simulink model "IEEE_1547_Testing"  (Simulink 9.2)
settings: Solver=ode4  StartTime=0.0  StopTime=inf  FixedStep=Ts  RelTol=1e-3  EnableMultiTasking=on
PreLoadFcn:
  | init_sandia
PostLoadFcn:
  | init_sandia
InitFcn:
  | init_sandia
values from neighbouring files (symbols this model uses):
  CURRENT_INPUT_OFFSET_PHA = 0    [init.m]    (also in init_sandia.m = 0.010681; init_sandia_hv.m = 0.010681)
  CURRENT_INPUT_OFFSET_PHB = 0    [init.m]    (also in init_sandia.m = 0.002978; init_sandia_hv.m = 0.002978)
  CURRENT_INPUT_OFFSET_PHC = 0    [init.m]    (also in init_sandia.m = 0.016506; init_sandia_hv.m = 0.016506)
  CURRENT_INPUT_SCALE_PHA = (1/0.03)*1.0002    (= 33.34)    [init.m]    (also in init_sandia.m = 93.940301; init_sandia_hv.m = 93.940301)
  CURRENT_INPUT_SCALE_PHB = (1/0.03)*0.9994    (= 33.3133333333)    [init.m]    (also in init_sandia.m = 94.382594; init_sandia_hv.m = 94.382594)
  CURRENT_INPUT_SCALE_PHC = (1/0.03)*0.9977    (= 33.2566666667)    [init.m]    (also in init_sandia.m = 93.670072; init_sandia_hv.m = 93.670072)
  ENABLE_PHA = 1    [init.m]    (also in init_sandia.m; init_sandia_hv.m)
  ENABLE_PHB = 1    [init.m]    (also in init_sandia.m; init_sandia_hv.m)
  ENABLE_PHC = 1    [init.m]    (also in init_sandia.m; init_sandia_hv.m)
  FNOM = 60.0    (= 60)    [init.m]    (also in init_sandia.m; init_sandia_hv.m)
  FREQUENCY = 60.0    (= 60)    [init.m]    (also in init_sandia.m; init_sandia_hv.m)
  FREQUENCY_MAX_LIMIT = 66.0    (= 66)    [init.m]    (also in init_sandia.m; init_sandia_hv.m)
  FREQUENCY_MIN_LIMIT = 56.0    (= 56)    [init.m]    (also in init_sandia.m; init_sandia_hv.m)
  FRT_CONDITION = [1 1 1 0 ]    [init.m]    (also in init_sandia.m; init_sandia_hv.m)
  FRT_END_TIMING = [0.2 0.3 0.4 0.5]    [init.m]    (also in init_sandia.m; init_sandia_hv.m)
  FRT_START_TIMING = [0.1 0.2 0.3 0.4]    [init.m]    (also in init_sandia.m; init_sandia_hv.m)
  FRT_VALUES = [59.0 56.0 55.0 33.0]    [init.m]    (also in init_sandia.m; init_sandia_hv.m)
  MODE = 1    [init.m]    (also in init_sandia.m = 3; init_sandia_hv.m = 3)
  PHASE_PHA = 0    [init_sandia.m]    (also in init_sandia_hv.m)
  PHASE_PHB = -120    [init_sandia.m]    (also in init_sandia_hv.m)
  PHASE_PHC = 120    [init_sandia.m]    (also in init_sandia_hv.m)
  RMS_ENABLE = 0    [init.m]    (also in init_sandia.m; init_sandia_hv.m)
  ROCOF_ENABLE = 0    [init.m]    (also in init_sandia.m; init_sandia_hv.m)
  ROCOF_INIT = 60    [init.m]    (also in init_sandia.m; init_sandia_hv.m)
  ROCOF_VALUE = 3    [init.m]    (also in init_sandia.m; init_sandia_hv.m)
  ROCOM_ENABLE = 1    [init.m]    (also in init_sandia.m; init_sandia_hv.m)
  ROCOM_END_TIME = 100    [init.m]    (also in init_sandia.m; init_sandia_hv.m)
  ROCOM_INIT = 1    [init.m]    (also in init_sandia.m; init_sandia_hv.m)
  ROCOM_START_TIME = 0    [init.m]    (also in init_sandia.m; init_sandia_hv.m)
  ROCOM_VALUE = 13.8    [init.m]    (also in init_sandia.m; init_sandia_hv.m)
  Ts = 40e-6    (= 4e-05)    [init.m]    (also in init_sandia.m; init_sandia_hv.m)
  VNOM = 1.0    (= 1)    [init.m]    (also in init_sandia.m = 277.2; init_sandia_hv.m = 277.2)
  VOLT_INPUT_OFFSET_PHA = 0    [init.m]    (also in init_sandia.m = 0.034058; init_sandia_hv.m = 0.034058)
  VOLT_INPUT_OFFSET_PHB = 0    [init.m]    (also in init_sandia.m = 0.06754; init_sandia_hv.m = 0.06754)
  VOLT_INPUT_OFFSET_PHC = 0    [init.m]    (also in init_sandia.m = 0.037741; init_sandia_hv.m = 0.037741)
  VOLT_INPUT_SCALE_PHA = 20    [init.m]    (also in init_sandia.m = 509.604013; init_sandia_hv.m = 509.604013)
  VOLT_INPUT_SCALE_PHB = 20    [init.m]    (also in init_sandia.m = 499.19708; init_sandia_hv.m = 499.19708)
  VOLT_INPUT_SCALE_PHC = 20    [init.m]    (also in init_sandia.m = 498.302881; init_sandia_hv.m = 498.302881)
  VOLT_OUTPUT_SCALE_PHA = 120.0*sqrt(2)    [init.m]    (also in init_sandia.m = 0.0235682300259; init_sandia_hv.m = 0.011784115013)
  VOLT_OUTPUT_SCALE_PHB = 120.0*sqrt(2)    [init.m]    (also in init_sandia.m = 0.0235682300259; init_sandia_hv.m = 0.011784115013)
  VOLT_OUTPUT_SCALE_PHC = 120.0*sqrt(2)    [init.m]    (also in init_sandia.m = 0.0235682300259; init_sandia_hv.m = 0.011784115013)
  VOLT_PHA = 1    [init_sandia.m]    (also in init_sandia_hv.m)
  VOLT_PHB = 1    [init_sandia.m]    (also in init_sandia_hv.m)
  VOLT_PHC = 1    [init_sandia.m]    (also in init_sandia_hv.m)
  VOLTAGE_MAX_LIMIT = 1.1    [init.m]    (also in init_sandia.m; init_sandia_hv.m = 1.2)
  VOLTAGE_MIN_LIMIT = 0.0    (= 0)    [init.m]    (also in init_sandia.m; init_sandia_hv.m)
  VRT_CONDITION = [0 1 0 1 0 1 0 1 -1 -1 -1 -1 -1 -1 -1 -1 -1 -1 -1 -1]+1    [init.m]    (also in init_sandia.m; init_sandia_hv.m)
  VRT_END_TIMING = [0.2 0.3 0.4 0.5 0.6 0.7 0.8 0.9 1 1.1 1.2 1.3 1.4 1.5 1.6 1.7 1.8 1.9 2 2.1]    [init.m]    (also in init_sandia.m; init_sandia_hv.m)
  VRT_PHA_ENABLE = 0    [init.m]    (also in init_sandia.m; init_sandia_hv.m)
  VRT_PHB_ENABLE = 0    [init.m]    (also in init_sandia.m; init_sandia_hv.m)
  VRT_PHC_ENABLE = 0    [init.m]    (also in init_sandia.m; init_sandia_hv.m)
  VRT_START_TIMING = [0.1 0.2 0.3 0.4 0.5 0.6 0.7 0.8 0.9 1 0.1 0.2 0.3 0.4 0.5 0.6 0.7 0.8 0.9 1]    [init.m]    (also in init_sandia.m; init_sandia_hv.m)
  VRT_VALUES = [1.2 0.94 0 0.5 0.7 0.88 0.94 0.88 0.94 1.1 1.2 0.94 0 0.5 0.7 0.88 0.94 0.88 0.94 1.1]    [init.m]    (also in init_sandia.m = [1.0 0.94 0 0.5 0.7 0.88 0.94 0.88 0.94 1.1 1.2 0.94 0 0.5 0; init_sandia_hv.m = [1.0 0.94 0 0.5 0.7 0.88 0.94 0.88 0.94 1.1 1.2 0.94 0 0.5 0)
  WAV_ENABLE = 1    [init.m]    (also in init_sandia.m; init_sandia_hv.m)
undefined symbols (not defined in the file or in its folder): DiscIntNeverNeededParam, magnitude
libraries: simulink x17, powerlib_meascontrol x13, rtlab x5, pePowerMeasurement x3, rtio_opalrt_common x3, powerlib x1
(part 1 of 2)
settings Model: ARTEMISmethode_block_infos=$$__separator__$$  Creator=DETLDAQ  LastModifiedBy=DETLDAQ  NumberOfSteps=10
settings DataIOCC: SignalLoggingSaveFormat=Dataset
settings OptimizationCC: BlockReduction=off  BooleanDataType=off  OptimizeBlockIOStorage=off  BufferReuse=off  GlobalBufferReuse=off  ExpressionFolding=off  LocalBlockOutputs=off  OptimizeDataStoreBuffers=off  BusAssignmentInplaceUpdate=off
settings DebuggingCC: SaveWithParameterizedLinksMsg=none  SignalResolutionControl=TryResolveAllWithWarning  MultiTaskDSMMsg=warning  MultiTaskCondExecSysMsg=none  FcnCallInpInsideContextMsg=error  UnderSpecifiedDimensionMsg=warning
settings HardwareCC: TargetBitPerPointer=64  TargetBitPerSizeT=64  TargetBitPerPtrDiffT=64  TargetLongLongMode=on  TargetIntDivRoundTo=Zero  TargetEndianess=LittleEndian  TargetWordSize=64  TargetHWDeviceType=MATLAB Host  ProdEqTarget=off
settings GRTTargetCC: GeneratePreprocessorConditionals=Use local settings  CombineOutputUpdateFcns=on  GRTInterface=off
settings ConfigComp: CovHtmlReporting=off
settings SimscapeCC: SimscapeNormalizeSystem=off

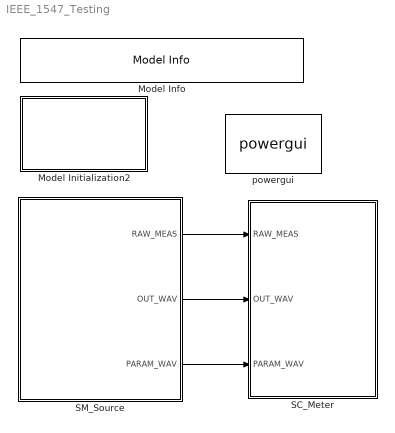
== system IEEE_1547_Testing ==
  Model Info : simulink/Model-Wide Utilities/Model Info  Frame=on  DisplayStringWithTags=|  HorizontalTextAlignment=Left  LeftAlignmentValue=0.02
      | %<ModelName>
      | 
      | - Verify that SVP drivers use model version : %<ModelVersion>
      | - Last modification:  %<LastModifiedBy> on %<LastModificationDate>
  Model Initialization2 : Subsystem  AncestorBlock=artemis/Tools /Misc/Model Initialization  mask(Model Functions){InitFcnX=init_sandia, prel=on, posl=on, inif=on, strf=off}
      mask prompts: InitFcnX "Initialisation"; prel "Preload Function"; posl "PostLoad Function"; inif "InitFcn"; strf "StartFcn"
      mask init:
      | currentBlock = gcb;
      | root = bdroot(currentBlock);
      | 
      | if ~strcmp(get_param(root,'BlockDiagramType'),'library')
      |     if prel==1
      |         set_param(root, 'PreLoadFcn', InitFcnX);
      |     else
      |         set_param(root, 'PreLoadFcn', '');
      |     end
      |     if inif==1
      |         set_param(root, 'InitFcn', InitFcnX);
      |     else
      |         set_param(root, 'InitFcn', '');
      |     end
      |     if strf==1
      |         set_param(root, 'StartFcn', InitFcnX);
      |     else
      |         set_param(root, 'StartFcn', '');
      |     end
      |     if posl==1
      |         set_param(root, 'PostLoadFcn', InitFcnX);
      |     else
      |         set_param(root, 'PostLoadFcn', '');
      |     end
      | end
      | 
      | pos = get_param(currentBlock, 'Position');
      | width = pos(3) - pos(1); height = pos(4) - pos(2);
      | txt = [ upper(root) '\n' '- InitFcn. . . . . '  get_param(root, 'InitFcn') ];
      settings: CopyFcn=set_param(gcb,'LinkStatus','inactive')
      mask Display: text(5, height*0.5, txt, 'horizontalAlignment', 'left', 'verticalAlignment', 'middle') ;
  SC_Meter : Subsystem
  SM_Source : Subsystem
  powergui : powerlib/powergui  Priority=1  SimulationMode=Discrete  SampleTime=Ts  frequency=60  Iterations=50  frequencyindice=0  Pbase=100e6  ErrMax=1e-4  UnitsV=kV  UnitsW=MW  buscounter=0  FunctionMessages=off  echomessages=off  EnableUseOfTLC=off  CurrentSourceSwitches=off  DisableSnubberDevices=off  DisableRonSwitches=off  DisableVfSwitches=off  DisplayEquations=off  SolverType=Backward Euler  Interpol=off  ExternalGateDelay=off  methode=off  Ts=100  x0status=blocks  SPID=off  SwTol=0  HookPort=off  RestoreLinks=warning  ResistiveCurrentMeasurement=off  Frange=[0:2:500]  Ylog=off  Xlog=on  ShowGrid=off  save=off  variable=ZData  structure=0  ZoomFFT=off  StartTime=0.0  cycles=1  DisplayStyle=1  fundamental=60  FreqAxis=off  MaxFrequency=1000  frequencyindicesteady=1  RmsSteady=1  display=off
  wires:
  SM_Source/1(RAW_MEAS) -> SC_Meter/1(RAW_MEAS)
  SM_Source/2(OUT_WAV) -> SC_Meter/2(OUT_WAV)
  SM_Source/3(PARAM_WAV) -> SC_Meter/3(PARAM_WAV)

== system IEEE_1547_Testing/Model Initialization2 ==

== system IEEE_1547_Testing/SC_Meter ==
  RAW_MEAS : Inport
  OUT_WAV : Inport  Port=2
  PARAM_WAV : Inport  Port=3
  Bus Selector : BusSelector  OutputSignals=voltage_pha,voltage_phb,voltage_phc,current_pha,current_phb,current_phc
  Bus Selector1 : BusSelector  OutputSignals=out_wav_pha,out_wav_phb,out_wav_phc
  Bus Selector2 : BusSelector  OutputSignals=wav_phase_pha,wav_phase_phb,wav_phase_phc,wav_voltage_pha,wav_voltage_phb,wav_voltage_phc,wav_frequency
  Mux{,1..4} (5 alike) : Mux  Inputs=3
  OpComm : rtlab/OpComm  nbport=3  groupe_acq=1  subsys_rate=Ts  st=0  Synchronization=on  Interpolation=on  Threshold=1.0  Missed_Data=off  Sim_Time=off  Samples=off  dynSigOut=off  from_console=0  warning_done=off  writeOpCommFile=off  Offset=off
      settings: SourceProductName=RT-LAB
  wires:
  RAW_MEAS/1 -> OpComm/1
  OUT_WAV/1 -> OpComm/2
  PARAM_WAV/1 -> OpComm/3
  OpComm/1 -> Bus Selector/1
  Bus Selector/1 -> Mux/1  "<voltage_pha>"
  Bus Selector/2 -> Mux/2  "<voltage_phb>"
  Bus Selector/3 -> Mux/3  "<voltage_phc>"
  Bus Selector/4 -> Mux1/1  "<current_pha>"
  Bus Selector/5 -> Mux1/2  "<current_phb>"
  Bus Selector/6 -> Mux1/3  "<current_phc>"
  OpComm/2 -> Bus Selector1/1
  Bus Selector1/2 -> Mux2/2  "<out_wav_phb>"
  Bus Selector1/3 -> Mux2/3  "<out_wav_phc>"
  Bus Selector1/1 -> Mux2/1  "<out_wav_pha>"
  OpComm/3 -> Bus Selector2/1
  Bus Selector2/1 -> Mux3/1  "<wav_phase_pha>"
  Bus Selector2/2 -> Mux3/2  "<wav_phase_phb>"
  Bus Selector2/3 -> Mux3/3  "<wav_phase_phc>"
  Bus Selector2/4 -> Mux4/1  "<wav_voltage_pha>"
  Bus Selector2/5 -> Mux4/2  "<wav_voltage_phb>"
  Bus Selector2/6 -> Mux4/3  "<wav_voltage_phc>"

== system IEEE_1547_Testing/SM_Source ==
  IEEE_1547_TESTING : Subsystem
  InputConnections : Subsystem
  OutputConnections : Subsystem
  RAW_MEAS : Outport
  OUT_WAV : Outport  Port=2
  PARAM_WAV : Outport  Port=3
  wires:
  InputConnections/1(RAW_MEAS (Nominal)) -> [RAW_MEAS], IEEE_1547_TESTING/1(RAW_MEAS (Nominal))
  [RAW_MEAS] -> RAW_MEAS/1
  [OUT_WAV] -> OUT_WAV/1
  IEEE_1547_TESTING/1(OUT_WAV (PU)) -> [OUT_WAV], OutputConnections/1(OUT_WAV (PU))
  IEEE_1547_TESTING/2(PARAM_WAV (PU)) -> [PARAM_WAV]
  [PARAM_WAV] -> PARAM_WAV/1

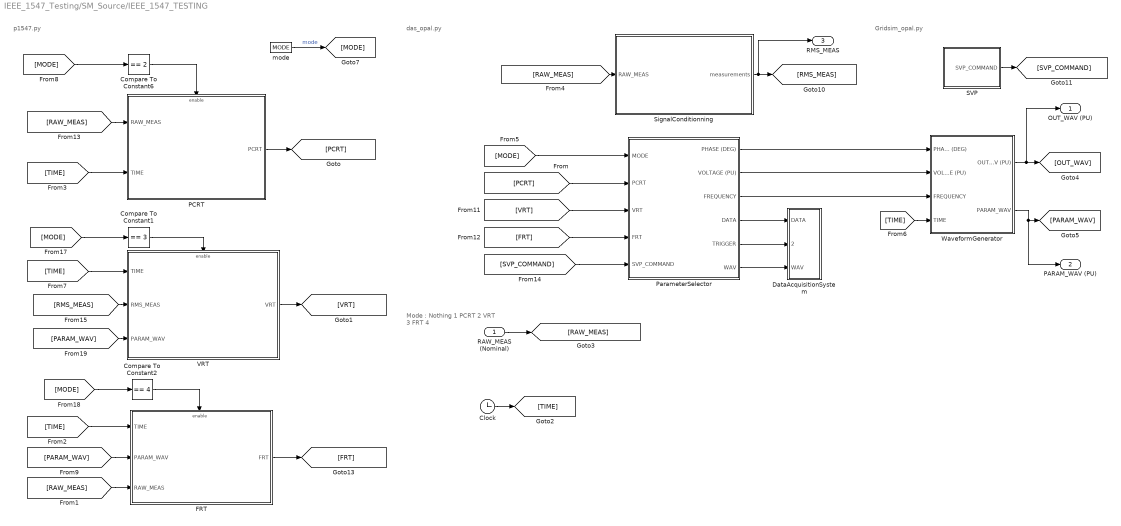
== system IEEE_1547_Testing/SM_Source/IEEE_1547_TESTING ==
  note: das_opal.py
  note: Gridsim_opal.py
  note: p1547.py
  note: Mode :
      |
      | Nothing
      | 1
      |
      | PCRT
      | 2
      |
      | VRT
      | 3
      |
      | FRT
      | 4
  RAW_MEAS (Nominal) : Inport
  Clock : Clock
  Compare To Constant1 : simulink/Logic and Bit Operations/Compare To Constant  relop===  const=3  OutDataTypeStr=boolean
  Compare To Constant2 : simulink/Logic and Bit Operations/Compare To Constant  relop===  const=4  OutDataTypeStr=boolean
  Compare To Constant6 : simulink/Logic and Bit Operations/Compare To Constant  relop===  const=2  OutDataTypeStr=boolean
  DataAcquisitionSystem : Subsystem
  FRT : Subsystem
  PCRT : Subsystem
  ParameterSelector : Subsystem
  SVP : Subsystem
  SignalConditionning : Subsystem
  VRT : Subsystem
  WaveformGenerator : Subsystem
  mode : Constant  Value=MODE
  OUT_WAV (PU) : Outport
  PARAM_WAV (PU) : Outport  Port=2
  RMS_MEAS : Outport  Port=3
  wires:
  mode/1 -> [MODE]  "mode"
  [RAW_MEAS] -> SignalConditionning/1(RAW_MEAS)
  [TIME] -> WaveformGenerator/4(TIME)
  ParameterSelector/5(TRIGGER) -> DataAcquisitionSystem/2(TRIGGER)
  ParameterSelector/1(PHASE (DEG)) -> WaveformGenerator/1(PHASE (DEG))
  SVP/1(SVP_COMMAND) -> [SVP_COMMAND]
  [SVP_COMMAND] -> ParameterSelector/5(SVP_COMMAND)
  [MODE] -> ParameterSelector/1(MODE)
  Clock/1 -> [TIME]
  [MODE] -> Compare To Constant6/1
  [RAW_MEAS] -> PCRT/1(RAW_MEAS)
  [FRT] -> ParameterSelector/4(FRT)
  ParameterSelector/4(DATA) -> DataAcquisitionSystem/1(DATA)
  ParameterSelector/2(VOLTAGE (PU)) -> WaveformGenerator/2(VOLTAGE (PU))
  [TIME] -> PCRT/2(TIME)
  [VRT] -> ParameterSelector/3(VRT)
  WaveformGenerator/1(OUT_WAV (PU)) -> OUT_WAV (PU)/1, [OUT_WAV]
  [PCRT] -> ParameterSelector/2(PCRT)
  [RMS_MEAS] -> VRT/2(RMS_MEAS)
  ParameterSelector/3(FREQUENCY) -> WaveformGenerator/3(FREQUENCY)
  PCRT/1(PCRT) -> [PCRT]
  Compare To Constant6/1 -> PCRT/Enable
  [MODE] -> Compare To Constant1/1
  VRT/1(VRT) -> [VRT]
  [MODE] -> Compare To Constant2/1
  WaveformGenerator/2(PARAM_WAV) -> PARAM_WAV (PU)/1, [PARAM_WAV]
  Compare To Constant1/1 -> VRT/Enable
  [PARAM_WAV] -> VRT/3(PARAM_WAV)
  RAW_MEAS (Nominal)/1 -> [RAW_MEAS]
  [TIME] -> VRT/1(TIME)
  [TIME] -> FRT/1(TIME)
  Compare To Constant2/1 -> FRT/Enable
  FRT/1(FRT) -> [FRT]
  [PARAM_WAV] -> FRT/2(PARAM_WAV)
  [RAW_MEAS] -> FRT/3(RAW_MEAS)
  ParameterSelector/6(WAV) -> DataAcquisitionSystem/3(WAV)
  SignalConditionning/1(measurements) -> RMS_MEAS/1, [RMS_MEAS]

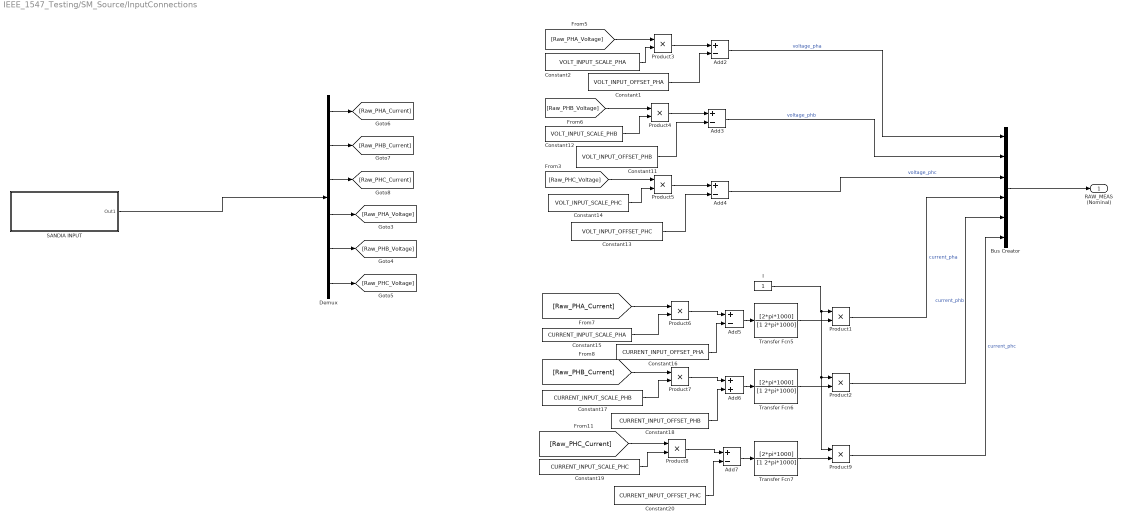
== system IEEE_1547_Testing/SM_Source/InputConnections ==
  Add{2..5,7} (5 alike) : Sum  Inputs=+-
  Add6 : Sum
  Bus Creator : BusCreator  Inputs=6
  Constant1 : Constant  Value=VOLT_INPUT_OFFSET_PHA
  Constant11 : Constant  Value=VOLT_INPUT_OFFSET_PHB
  Constant12 : Constant  Value=VOLT_INPUT_SCALE_PHB
  Constant13 : Constant  Value=VOLT_INPUT_OFFSET_PHC
  Constant14 : Constant  Value=VOLT_INPUT_SCALE_PHC
  Constant15 : Constant  Value=CURRENT_INPUT_SCALE_PHA
  Constant16 : Constant  Value=CURRENT_INPUT_OFFSET_PHA
  Constant17 : Constant  Value=CURRENT_INPUT_SCALE_PHB
  Constant18 : Constant  Value=CURRENT_INPUT_OFFSET_PHB
  Constant19 : Constant  Value=CURRENT_INPUT_SCALE_PHC
  Constant2 : Constant  Value=VOLT_INPUT_SCALE_PHA
  Constant20 : Constant  Value=CURRENT_INPUT_OFFSET_PHC
  Demux : Demux  Outputs=6
  I : Constant
  Product{1..9} (9 alike) : Product
  SANDIA INPUT : Subsystem
  Transfer Fcn5 : TransferFcn  Numerator=[2*pi*1000]  Denominator=[1 2*pi*1000]
  Transfer Fcn6 : TransferFcn  Numerator=[2*pi*1000]  Denominator=[1 2*pi*1000]
  Transfer Fcn7 : TransferFcn  Numerator=[2*pi*1000]  Denominator=[1 2*pi*1000]
  RAW_MEAS (Nominal) : Outport
  wires:
  [Raw_PHB_Current] -> Product7/1
  Product6/1 -> Add5/1
  Constant17/1 -> Product7/2
  I/1 -> Product9/1, Product2/1, Product1/1
  Transfer Fcn6/1 -> Product2/2
  Constant14/1 -> Product5/2
  Constant13/1 -> Add4/2
  [Raw_PHB_Voltage] -> Product4/1
  Product8/1 -> Add7/1
  Product5/1 -> Add4/1
  Constant15/1 -> Product6/2
  [Raw_PHC_Voltage] -> Product5/1
  Constant20/1 -> Add7/2
  Add6/1 -> Transfer Fcn6/1
  Add5/1 -> Transfer Fcn5/1
  Product7/1 -> Add6/1
  [Raw_PHA_Voltage] -> Product3/1
  Constant18/1 -> Add6/2
  [Raw_PHA_Current] -> Product6/1
  Transfer Fcn7/1 -> Product9/2
  [Raw_PHC_Current] -> Product8/1
  Add7/1 -> Transfer Fcn7/1
  Constant16/1 -> Add5/2
  Transfer Fcn5/1 -> Product1/2
  Product4/1 -> Add3/1
  Product3/1 -> Add2/1
  Constant19/1 -> Product8/2
  Add2/1 -> Bus Creator/1  "voltage_pha"
  Add3/1 -> Bus Creator/2  "voltage_phb"
  Add4/1 -> Bus Creator/3  "voltage_phc"
  Product1/1 -> Bus Creator/4  "current_pha"
  Product2/1 -> Bus Creator/5  "current_phb"
  Product9/1 -> Bus Creator/6  "current_phc"
  Bus Creator/1 -> RAW_MEAS (Nominal)/1
  Constant2/1 -> Product3/2
  Constant11/1 -> Add3/2
  Constant12/1 -> Product4/2
  Constant1/1 -> Add2/2
  Demux/1 -> [Raw_PHA_Current]
  Demux/2 -> [Raw_PHB_Current]
  Demux/3 -> [Raw_PHC_Current]
  Demux/4 -> [Raw_PHA_Voltage]
  Demux/5 -> [Raw_PHB_Voltage]
  Demux/6 -> [Raw_PHC_Voltage]
  SANDIA INPUT/1(Out1) -> Demux/1

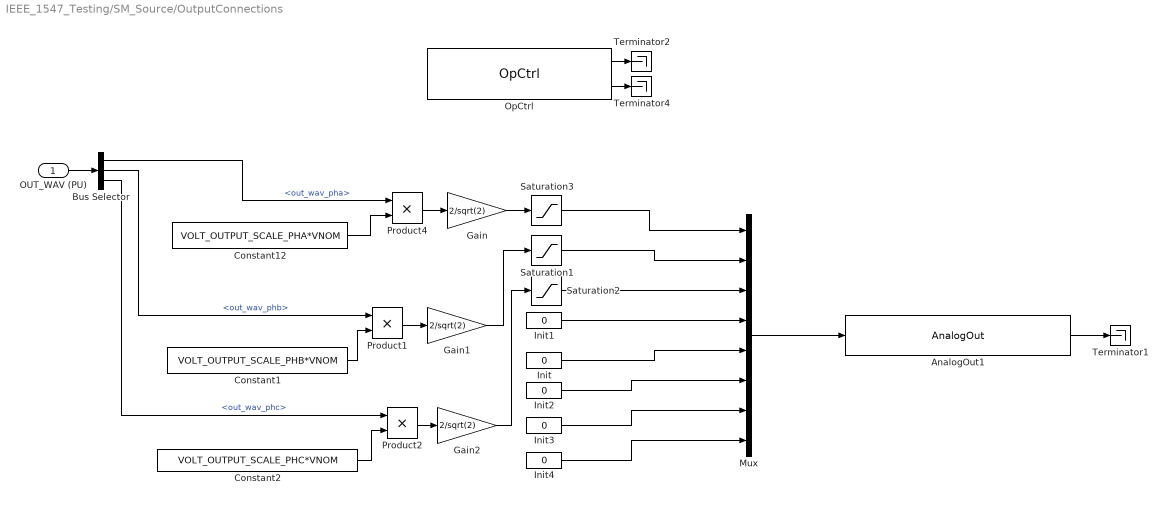
== system IEEE_1547_Testing/SM_Source/OutputConnections ==
  OUT_WAV (PU) : Inport
  AnalogOut1 : rtio_opalrt_common/AnalogOut  CtrlName='OpCtrl'  portNb=1  FcnNos=Slot 1 Module A Subsection 1  size=16  maxcount=8  count=8  numchan=8  israngeinput=off  voltagerange=[-16 ... 16]  slot=0  side=0  mismatch=0  slotside=Slot_1_Module_A
      settings: AttributesFormatString=%<CtrlName>
  Bus Selector : BusSelector  OutputSignals=out_wav_pha,out_wav_phb,out_wav_phc
  Constant1 : Constant  Value=VOLT_OUTPUT_SCALE_PHB*VNOM
  Constant12 : Constant  Value=VOLT_OUTPUT_SCALE_PHA*VNOM
  Constant2 : Constant  Value=VOLT_OUTPUT_SCALE_PHC*VNOM
  Gain : Gain  Gain=2/sqrt(2)
  Gain1 : Gain  Gain=2/sqrt(2)
  Gain2 : Gain  Gain=2/sqrt(2)
  Init{,1..4} (5 alike) : Constant  Value=0
  Mux : Mux  Inputs=8
  OpCtrl : rtio_opalrt_common/OpCtrl  CtrlName='OpCtrl'  boardid=0  BitstreamFilename=ML605_2-EX-0029-2_3_7_140-32Ao_16Ai_32DioSelectable_C3C1C3FBFBEA-01-05.bin  numconfig=-1  mode=Master  externalClock=off  decimRtsi=0  calibIO=off  SampleTime=0  loadinport=-1  BoardType=ML605  SecondaryPresent=off  sync_type=Audio  scope_enable=off  scope_acqPeriodSec=0  scope_trigPos=0
  Product1 : Product
  Product2 : Product
  Product4 : Product
  Saturation1 : Saturate  UpperLimit=15  LowerLimit=-15
  Saturation2 : Saturate  UpperLimit=15  LowerLimit=-15
  Saturation3 : Saturate  UpperLimit=15  LowerLimit=-15
  Terminator1 : Terminator
  Terminator2 : Terminator
  Terminator4 : Terminator
  wires:
  OUT_WAV (PU)/1 -> Bus Selector/1
  Product4/1 -> Gain/1
  Constant12/1 -> Product4/2
  Bus Selector/1 -> Product4/1  "<out_wav_pha>"
  Constant1/1 -> Product1/2
  Bus Selector/2 -> Product1/1  "<out_wav_phb>"
  Constant2/1 -> Product2/2
  Bus Selector/3 -> Product2/1  "<out_wav_phc>"
  Saturation2/1 -> Mux/3
  Saturation3/1 -> Mux/1
  Saturation1/1 -> Mux/2
  Mux/1 -> AnalogOut1/1
  Init/1 -> Mux/5
  Init1/1 -> Mux/4
  Init2/1 -> Mux/6
  Init3/1 -> Mux/7
  Init4/1 -> Mux/8
  OpCtrl/1 -> Terminator2/1
  OpCtrl/2 -> Terminator4/1
  AnalogOut1/1 -> Terminator1/1
  Gain/1 -> Saturation3/1
  Product2/1 -> Gain2/1
  Gain2/1 -> Saturation2/1
  Product1/1 -> Gain1/1
  Gain1/1 -> Saturation1/1

== system IEEE_1547_Testing/SM_Source/IEEE_1547_TESTING/DataAcquisitionSystem ==
  DATA : Inport
  TRIGGER : Inport  Port=2
  WAV : Inport  Port=3
  Compare To Constant1 : simulink/Logic and Bit Operations/Compare To Constant  relop===  const=1  OutDataTypeStr=boolean
  Compare To Constant2 : simulink/Logic and Bit Operations/Compare To Constant  relop===  const=1  OutDataTypeStr=boolean
  Constant : Constant  Value=RMS_ENABLE
  Constant1 : Constant  Value=WAV_ENABLE
  OpTrigger : rtlab/DataLogging/OpTrigger  Trig_Type=TRIGGER SIGNAL >= TRIGGER LEVEL  Trig_Offset=-(1/Ts)  Acq_Group=28
      settings: SourceProductName=RT-LAB
  OpTrigger1 : rtlab/DataLogging/OpTrigger  Trig_Type=TRIGGER SIGNAL >= TRIGGER LEVEL  Trig_Offset=0  Acq_Group=27
      settings: SourceProductName=RT-LAB
  Subsystem : Subsystem
  Subsystem1 : Subsystem
  TRIGGER_STATUS : Gain
  TRIGGER_STATUS1 : Gain
  Terminator2 : Terminator
  Terminator3 : Terminator
  Trigger_level : Constant
  wires:
  OpTrigger/1 -> TRIGGER_STATUS/1
  Trigger_level/1 -> OpTrigger/2, OpTrigger1/2
  TRIGGER_STATUS/1 -> Terminator2/1
  TRIGGER_STATUS1/1 -> Terminator3/1
  OpTrigger1/1 -> TRIGGER_STATUS1/1
  TRIGGER/1 -> OpTrigger1/1, OpTrigger/1
  DATA/1 -> Subsystem/1(In1)
  Constant/1 -> Compare To Constant1/1
  Compare To Constant1/1 -> Subsystem/Enable
  Constant1/1 -> Compare To Constant2/1
  Compare To Constant2/1 -> Subsystem1/Enable
  WAV/1 -> Subsystem1/1(In1)

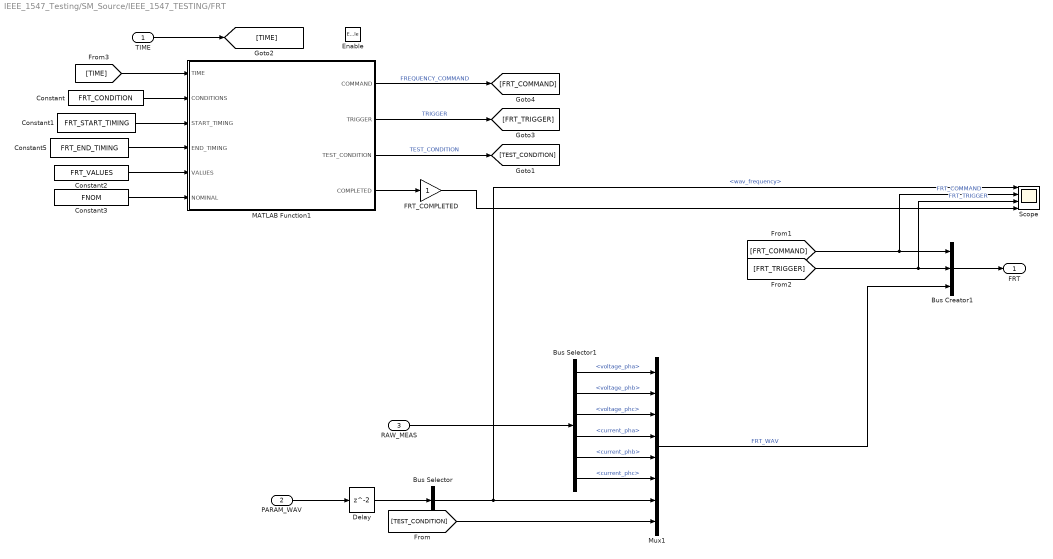
== system IEEE_1547_Testing/SM_Source/IEEE_1547_TESTING/FRT ==
  TIME : Inport
  PARAM_WAV : Inport  Port=2
  RAW_MEAS : Inport  Port=3
  Enable : EnablePort
  Bus Creator1 : BusCreator  Inputs=3
  Bus Selector : BusSelector  OutputSignals=wav_frequency
  Bus Selector1 : BusSelector  OutputSignals=voltage_pha,voltage_phb,voltage_phc,current_pha,current_phb,current_phc
  Constant : Constant  Value=FRT_CONDITION
  Constant1 : Constant  Value=FRT_START_TIMING
  Constant2 : Constant  Value=FRT_VALUES
  Constant3 : Constant  Value=FNOM
  Constant5 : Constant  Value=FRT_END_TIMING
  Delay : Delay
  FRT_COMPLETED : Gain
  MATLAB Function1 : MATLAB Function  TreatAsAtomicUnit=on
  Mux1 : Mux  Inputs=8
  Scope : Scope  NumInputPorts=4
  FRT : Outport  VectorParamsAs1DForOutWhenUnconnected=on
  wires:
  Mux1/1 -> Bus Creator1/3  "FRT_WAV"
  MATLAB Function1/1(COMMAND) -> [FRT_COMMAND]  "FREQUENCY_COMMAND"
  MATLAB Function1/3(TEST_CONDITION) -> [TEST_CONDITION]  "TEST_CONDITION"
  [TIME] -> MATLAB Function1/1(TIME)
  [FRT_TRIGGER] -> Scope/3, Bus Creator1/2  "FRT_TRIGGER"
  Constant/1 -> MATLAB Function1/2(CONDITIONS)
  TIME/1 -> [TIME]
  Constant2/1 -> MATLAB Function1/5(VALUES)
  Constant5/1 -> MATLAB Function1/4(END_TIMING)
  MATLAB Function1/2(TRIGGER) -> [FRT_TRIGGER]  "TRIGGER"
  PARAM_WAV/1 -> Delay/1
  Bus Creator1/1 -> FRT/1
  MATLAB Function1/4(COMPLETED) -> FRT_COMPLETED/1
  Constant1/1 -> MATLAB Function1/3(START_TIMING)
  [FRT_COMMAND] -> Scope/2, Bus Creator1/1  "FRT_COMMAND"
  [TEST_CONDITION] -> Mux1/8
  Delay/1 -> Bus Selector/1
  Bus Selector/1 -> Scope/1, Mux1/7  "<wav_frequency>"
  RAW_MEAS/1 -> Bus Selector1/1
  Bus Selector1/1 -> Mux1/1  "<voltage_pha>"
  Bus Selector1/2 -> Mux1/2  "<voltage_phb>"
  Bus Selector1/3 -> Mux1/3  "<voltage_phc>"
  Constant3/1 -> MATLAB Function1/6(NOMINAL)
  FRT_COMPLETED/1 -> Scope/4
  Bus Selector1/4 -> Mux1/4  "<current_pha>"
  Bus Selector1/5 -> Mux1/5  "<current_phb>"
  Bus Selector1/6 -> Mux1/6  "<current_phc>"

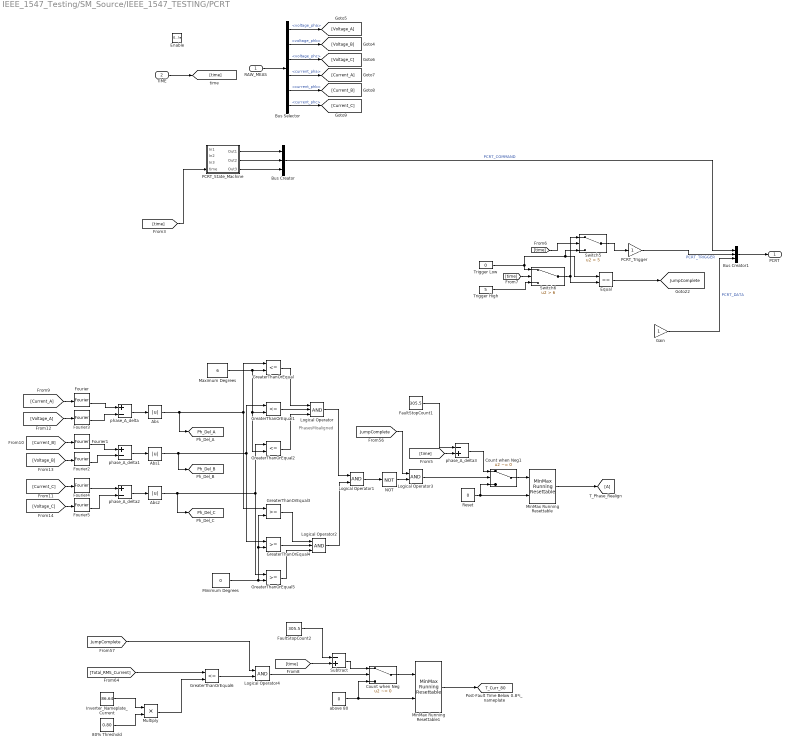
== system IEEE_1547_Testing/SM_Source/IEEE_1547_TESTING/PCRT ==
  note: PhasesMisaligned
  RAW_MEAS : Inport
  TIME : Inport  Port=2
  Enable : EnablePort
  80% Threshold : Constant  Value=0.80
  Abs : Abs
  Abs1 : Abs
  Abs2 : Abs
  Bus Creator : BusCreator  Inputs=3
  Bus Creator1 : BusCreator  Inputs=3
  Bus Selector : BusSelector  OutputSignals=voltage_pha,voltage_phb,voltage_phc,current_pha,current_phb,current_phc
  Count when Neg : Switch  Criteria=u2 ~= 0
  Count when Neg1 : Switch  Criteria=u2 ~= 0
  Equal : RelationalOperator  Operator===  OutDataTypeStr=boolean  RndMeth=Simplest
  FaultStopCount1 : Constant  Value=305.5
  FaultStopCount2 : Constant  Value=305.5
  Fourier{,1..5} (6 alike) : powerlib_meascontrol/Measurements/Fourier  Freq=60  n=1  InInit=[0, 0]  Ts=0
  Gain : Gain
  GreaterThanOrEqual{,1..2,6} (4 alike) : RelationalOperator  Operator=<=  OutDataTypeStr=boolean  RndMeth=Simplest
  GreaterThanOrEqual3 : RelationalOperator  OutDataTypeStr=boolean  RndMeth=Simplest
  GreaterThanOrEqual4 : RelationalOperator  OutDataTypeStr=boolean  RndMeth=Simplest
  GreaterThanOrEqual5 : RelationalOperator  OutDataTypeStr=boolean  RndMeth=Simplest
  Inverter_Nameplate_Current : Constant  Value=86.64
  Logical Operator : Logic  Inputs=3  AllPortsSameDT=off  OutDataTypeStr=boolean
  Logical Operator1 : Logic  AllPortsSameDT=off  OutDataTypeStr=boolean
  Logical Operator2 : Logic  Inputs=3  AllPortsSameDT=off  OutDataTypeStr=boolean
  Logical Operator3 : Logic  AllPortsSameDT=off  OutDataTypeStr=boolean
  Logical Operator4 : Logic  AllPortsSameDT=off  OutDataTypeStr=boolean
  Maximum Degrees : Constant  Value=6
  MinMax Running Resettable : simulink/Math Operations/MinMax Running Resettable  Function=max  vinit=0.0
  MinMax Running Resettable1 : simulink/Math Operations/MinMax Running Resettable  Function=max  vinit=0.0
  Minimum Degrees : Constant  Value=0
  Multiply : Product
  NOT : Logic  Operator=NOT  IconShape=distinctive  AllPortsSameDT=off  OutDataTypeStr=boolean
  PCRT_State_Machine : Subsystem
  PCRT_Trigger : Gain
  Reset : Constant  Value=0
  Subtract : Sum  Inputs=-+
  Switch5 : Switch  Criteria=u2 > Threshold  Threshold=5
  Switch6 : Switch  Criteria=u2 > Threshold  Threshold=6
  Trigger High : Constant  Value=5
  Trigger Low : Constant  Value=0
  above 80 : Constant  Value=0
  phase_A_delta : Sum  Inputs=+-
  phase_A_delta1 : Sum  Inputs=+-
  phase_A_delta2 : Sum  Inputs=+-
  phase_A_delta3 : Sum  Inputs=-+
  PCRT : Outport  VectorParamsAs1DForOutWhenUnconnected=on
  tag scope: JumpComplete=global, Ph_Del_A=global, Ph_Del_B=global, Ph_Del_C=global, T_Curr_80=global
  wires:
  Abs/1 -> GreaterThanOrEqual/1, GreaterThanOrEqual3/1, [Ph_Del_A]
  Abs2/1 -> GreaterThanOrEqual2/1, GreaterThanOrEqual5/1, [Ph_Del_C]
  phase_A_delta2/1 -> Abs2/1
  Abs1/1 -> GreaterThanOrEqual1/1, GreaterThanOrEqual4/1, [Ph_Del_B]
  GreaterThanOrEqual5/1 -> Logical Operator2/3
  Minimum Degrees/1 -> GreaterThanOrEqual3/2, GreaterThanOrEqual4/2, GreaterThanOrEqual5/2
  GreaterThanOrEqual/1 -> Logical Operator/1
  Reset/1 -> MinMax Running Resettable/2, Count when Neg1/3
  GreaterThanOrEqual4/1 -> Logical Operator2/2
  GreaterThanOrEqual3/1 -> Logical Operator2/1
  Logical Operator3/1 -> Count when Neg1/2
  NOT/1 -> Logical Operator3/2
  Logical Operator/1 -> Logical Operator1/1
  Fourier3/2 -> phase_A_delta/2
  Logical Operator2/1 -> Logical Operator1/2
  Logical Operator1/1 -> NOT/1
  GreaterThanOrEqual1/1 -> Logical Operator/2
  [time] -> phase_A_delta3/2
  FaultStopCount1/1 -> phase_A_delta3/1
  Maximum Degrees/1 -> GreaterThanOrEqual/2, GreaterThanOrEqual2/2, GreaterThanOrEqual1/2
  [JumpComplete] -> Logical Operator3/1
  phase_A_delta3/1 -> Count when Neg1/1
  phase_A_delta/1 -> Abs/1
  Fourier/2 -> phase_A_delta/1
  Count when Neg1/1 -> MinMax Running Resettable/1
  Fourier5/2 -> phase_A_delta2/2
  phase_A_delta1/1 -> Abs1/1
  Fourier4/2 -> phase_A_delta2/1
  GreaterThanOrEqual2/1 -> Logical Operator/3
  Fourier1/2 -> phase_A_delta1/1
  Fourier2/2 -> phase_A_delta1/2
  RAW_MEAS/1 -> Bus Selector/1
  Trigger High/1 -> Switch6/3
  Equal/1 -> [JumpComplete]
  [time] -> Switch6/2
  Trigger Low/1 -> Equal/1, Switch5/3, Switch6/1
  Switch6/1 -> Equal/2, Switch5/1
  [time] -> Switch5/2
  Switch5/1 -> PCRT_Trigger/1
  TIME/1 -> [time]
  [time] -> Subtract/2
  FaultStopCount2/1 -> Subtract/1
  [JumpComplete] -> Logical Operator4/1
  Subtract/1 -> Count when Neg/1
  Multiply/1 -> GreaterThanOrEqual6/2
  Count when Neg/1 -> MinMax Running Resettable1/1
  above 80/1 -> Count when Neg/3, MinMax Running Resettable1/2
  Inverter_Nameplate_Current/1 -> Multiply/1
  [Total_RMS_Current] -> GreaterThanOrEqual6/1
  Logical Operator4/1 -> Count when Neg/2
  GreaterThanOrEqual6/1 -> Logical Operator4/2
  MinMax Running Resettable1/1 -> [T_Curr_80]
  80% Threshold/1 -> Multiply/2
  PCRT_State_Machine/1(Out1) -> Bus Creator/1
  PCRT_State_Machine/2(Out2) -> Bus Creator/2
  PCRT_State_Machine/3(Out3) -> Bus Creator/3
  [time] -> PCRT_State_Machine/4(time)
  Bus Selector/1 -> [Voltage_A]  "<voltage_pha>"
  Bus Selector/2 -> [Voltage_B]  "<voltage_phb>"
  Bus Selector/3 -> [Voltage_C]  "<voltage_phc>"
  Bus Selector/4 -> [Current_A]  "<current_pha>"
  Bus Selector/5 -> [Current_B]  "<current_phb>"
  Bus Selector/6 -> [Current_C]  "<current_phc>"
  [Current_A] -> Fourier/1
  [Current_C] -> Fourier4/1
  [Current_B] -> Fourier1/1
  [Voltage_A] -> Fourier3/1
  [Voltage_B] -> Fourier2/1
  [Voltage_C] -> Fourier5/1
  MinMax Running Resettable/1 -> [A]
  Gain/1 -> Bus Creator1/3  "PCRT_DATA"
  PCRT_Trigger/1 -> Bus Creator1/2  "PCRT_TRIGGER"
  Bus Creator/1 -> Bus Creator1/1  "PCRT_COMMAND"
  Bus Creator1/1 -> PCRT/1

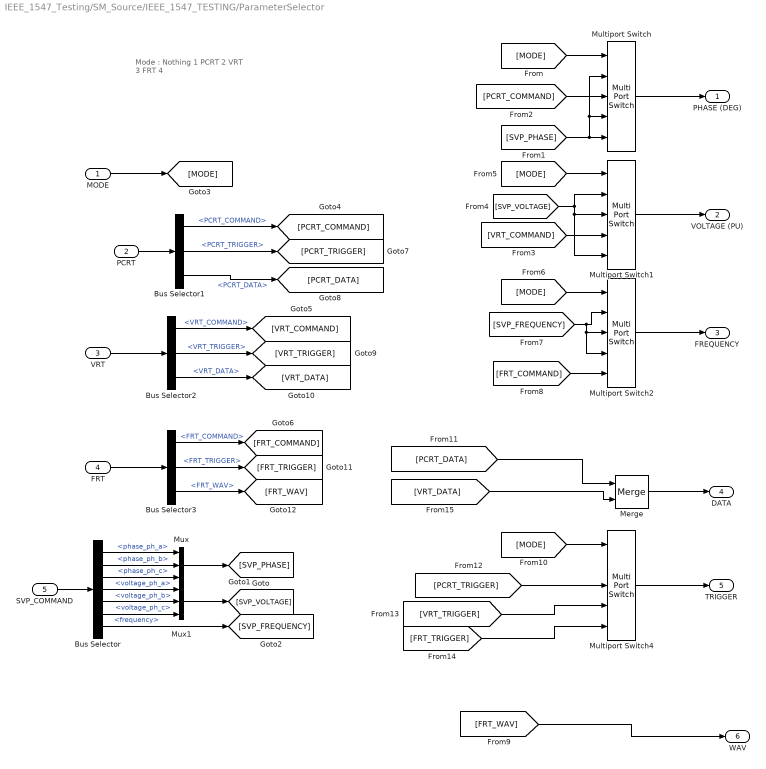
== system IEEE_1547_Testing/SM_Source/IEEE_1547_TESTING/ParameterSelector ==
  note: Mode :
      |
      | Nothing
      | 1
      |
      | PCRT
      | 2
      |
      | VRT
      | 3
      |
      | FRT
      | 4
  MODE : Inport
  PCRT : Inport  Port=2
  VRT : Inport  Port=3
  FRT : Inport  Port=4
  SVP_COMMAND : Inport  Port=5
  Bus Selector : BusSelector  OutputSignals=phase_ph_a,phase_ph_b,phase_ph_c,voltage_ph_a,voltage_ph_b,voltage_ph_c,frequency
  Bus Selector1 : BusSelector  OutputSignals=PCRT_COMMAND,PCRT_TRIGGER,PCRT_DATA
  Bus Selector2 : BusSelector  OutputSignals=VRT_COMMAND,VRT_TRIGGER,VRT_DATA
  Bus Selector3 : BusSelector  OutputSignals=FRT_COMMAND,FRT_TRIGGER,FRT_WAV
  Merge : Merge  AllowUnequalInputPortWidths=on
  Multiport Switch{,1..2,4} (4 alike) : MultiPortSwitch  Inputs=4
  Mux : Mux  Inputs=3
  Mux1 : Mux  Inputs=3
  PHASE (DEG) : Outport  VectorParamsAs1DForOutWhenUnconnected=on
  VOLTAGE (PU) : Outport  Port=2  VectorParamsAs1DForOutWhenUnconnected=on
  FREQUENCY : Outport  Port=3  VectorParamsAs1DForOutWhenUnconnected=on
  DATA : Outport  Port=4  VectorParamsAs1DForOutWhenUnconnected=on
  TRIGGER : Outport  Port=5  VectorParamsAs1DForOutWhenUnconnected=on
  WAV : Outport  Port=6  VectorParamsAs1DForOutWhenUnconnected=on
  wires:
  SVP_COMMAND/1 -> Bus Selector/1
  Bus Selector/2 -> Mux/2  "<phase_ph_b>"
  Bus Selector/1 -> Mux/1  "<phase_ph_a>"
  Bus Selector/3 -> Mux/3  "<phase_ph_c>"
  Bus Selector/4 -> Mux1/1  "<voltage_ph_a>"
  Bus Selector/5 -> Mux1/2  "<voltage_ph_b>"
  Bus Selector/6 -> Mux1/3  "<voltage_ph_c>"
  Mux/1 -> [SVP_PHASE]
  Mux1/1 -> [SVP_VOLTAGE]
  Bus Selector/7 -> [SVP_FREQUENCY]  "<frequency>"
  MODE/1 -> [MODE]
  [MODE] -> Multiport Switch/1
  [PCRT_COMMAND] -> Multiport Switch/3
  [SVP_PHASE] -> Multiport Switch/2, Multiport Switch/4, Multiport Switch/5
  Multiport Switch/1 -> PHASE (DEG)/1
  Multiport Switch1/1 -> VOLTAGE (PU)/1
  Multiport Switch2/1 -> FREQUENCY/1
  [VRT_COMMAND] -> Multiport Switch1/4
  [SVP_VOLTAGE] -> Multiport Switch1/3, Multiport Switch1/5, Multiport Switch1/2
  [MODE] -> Multiport Switch1/1
  [MODE] -> Multiport Switch2/1
  [SVP_FREQUENCY] -> Multiport Switch2/3, Multiport Switch2/4, Multiport Switch2/2
  [FRT_COMMAND] -> Multiport Switch2/5
  PCRT/1 -> Bus Selector1/1
  Bus Selector1/1 -> [PCRT_COMMAND]  "<PCRT_COMMAND>"
  Bus Selector1/2 -> [PCRT_TRIGGER]  "<PCRT_TRIGGER>"
  Bus Selector1/3 -> [PCRT_DATA]  "<PCRT_DATA>"
  Merge/1 -> DATA/1
  Multiport Switch4/1 -> TRIGGER/1
  VRT/1 -> Bus Selector2/1
  Bus Selector2/1 -> [VRT_COMMAND]  "<VRT_COMMAND>"
  Bus Selector2/2 -> [VRT_TRIGGER]  "<VRT_TRIGGER>"
  Bus Selector2/3 -> [VRT_DATA]  "<VRT_DATA>"
  FRT/1 -> Bus Selector3/1
  Bus Selector3/1 -> [FRT_COMMAND]  "<FRT_COMMAND>"
  Bus Selector3/2 -> [FRT_TRIGGER]  "<FRT_TRIGGER>"
  Bus Selector3/3 -> [FRT_WAV]  "<FRT_WAV>"
  [MODE] -> Multiport Switch4/1
  [PCRT_TRIGGER] -> Multiport Switch4/3
  [PCRT_DATA] -> Merge/1
  [VRT_TRIGGER] -> Multiport Switch4/4
  [FRT_TRIGGER] -> Multiport Switch4/5
  [VRT_DATA] -> Merge/2
  [FRT_WAV] -> WAV/1

== system IEEE_1547_Testing/SM_Source/IEEE_1547_TESTING/SVP ==
  Bus Creator : BusCreator  Inputs=7
  Constant : Constant  Value=FREQUENCY
  phase_pha : Constant  Value=PHASE_PHA
  phase_phb : Constant  Value=PHASE_PHB
  phase_phc : Constant  Value=PHASE_PHC
  voltage_ph_a : Constant  Value=VOLT_PHA
  voltage_ph_b : Constant  Value=VOLT_PHB
  voltage_ph_c : Constant  Value=VOLT_PHC
  SVP_COMMAND : Outport
  wires:
  phase_phb/1 -> Bus Creator/2  "phase_ph_b"
  phase_phc/1 -> Bus Creator/3  "phase_ph_c"
  phase_pha/1 -> Bus Creator/1  "phase_ph_a"
  voltage_ph_a/1 -> Bus Creator/4  "voltage_ph_a"
  voltage_ph_c/1 -> Bus Creator/6  "voltage_ph_c"
  voltage_ph_b/1 -> Bus Creator/5  "voltage_ph_b"
  Constant/1 -> Bus Creator/7  "frequency"
  Bus Creator/1 -> SVP_COMMAND/1

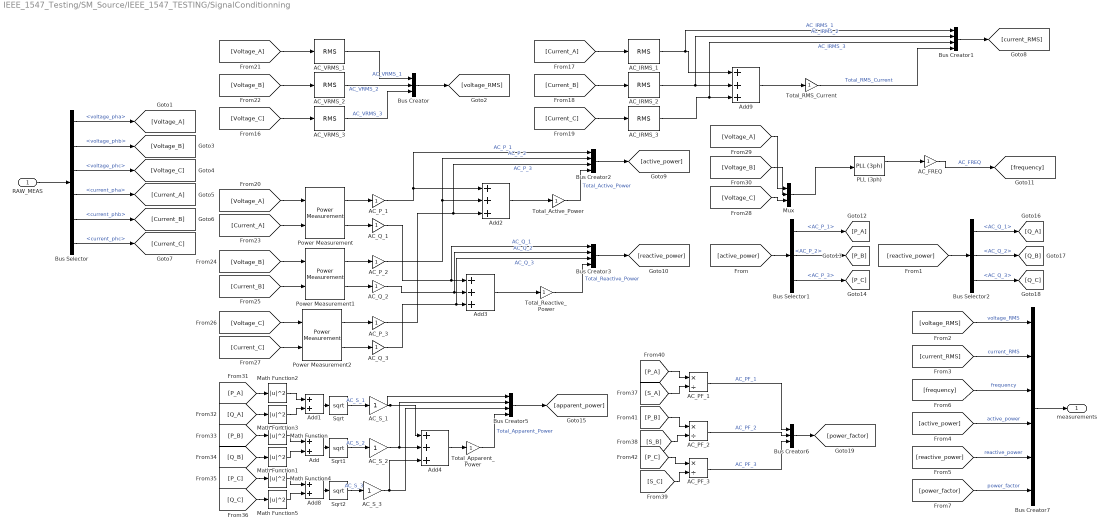
== system IEEE_1547_Testing/SM_Source/IEEE_1547_TESTING/SignalConditionning ==
  RAW_MEAS : Inport
  AC_FREQ : Gain
  AC_IRMS_1 : powerlib_meascontrol/Measurements/RMS  TrueRMS=on  Freq=60  RMSInit=120  Ts=0
  AC_IRMS_2 : powerlib_meascontrol/Measurements/RMS  TrueRMS=on  Freq=60  RMSInit=120  Ts=0
  AC_IRMS_3 : powerlib_meascontrol/Measurements/RMS  TrueRMS=on  Freq=60  RMSInit=120  Ts=0
  AC_PF_1 : Product  Inputs=*/
  AC_PF_2 : Product  Inputs=*/
  AC_PF_3 : Product  Inputs=*/
  AC_P_1 : Gain
  AC_P_2 : Gain
  AC_P_3 : Gain
  AC_Q_1 : Gain
  AC_Q_2 : Gain
  AC_Q_3 : Gain
  AC_S_1 : Gain
  AC_S_2 : Gain
  AC_S_3 : Gain
  AC_VRMS_1 : powerlib_meascontrol/Measurements/RMS  TrueRMS=on  Freq=60  RMSInit=120  Ts=0
  AC_VRMS_2 : powerlib_meascontrol/Measurements/RMS  TrueRMS=on  Freq=60  RMSInit=120  Ts=0
  AC_VRMS_3 : powerlib_meascontrol/Measurements/RMS  TrueRMS=on  Freq=60  RMSInit=120  Ts=0
  Add : Sum
  Add1 : Sum
  Add{2..4,9} (4 alike) : Sum  Inputs=+++
  Add8 : Sum
  Bus Creator : BusCreator  Inputs=3
  Bus Creator{1..3,5} (4 alike) : BusCreator  Inputs=4
  Bus Creator6 : BusCreator  Inputs=3
  Bus Creator7 : BusCreator  Inputs=6
  Bus Selector : BusSelector  OutputSignals=voltage_pha,voltage_phb,voltage_phc,current_pha,current_phb,current_phc
  Bus Selector1 : BusSelector  OutputSignals=AC_P_1,AC_P_2,AC_P_3
  Bus Selector2 : BusSelector  OutputSignals=AC_Q_1,AC_Q_2,AC_Q_3
  Math Function{,1..5} (6 alike) : Math  Operator=magnitude^2  SaturateOnIntegerOverflow=on
  Mux : Mux  Inputs=3
  PLL (3ph) : powerlib_meascontrol/PLL/PLL (3ph)  Fmin=50  Par_Init=[0, 60]  ParK=[180, 3200, 1]  TcD=1e-4  MaxRateChangeFreq=5  FilterCutOffFreq=25  Ts=Ts  AGC=on
  Power Measurement : pePowerMeasurement/Power Measurement  LabelModeActiveChoice=Continuous  F=60  K=1  Ts=0
  Power Measurement1 : pePowerMeasurement/Power Measurement  LabelModeActiveChoice=Continuous  F=60  K=1  Ts=0
  Power Measurement2 : pePowerMeasurement/Power Measurement  LabelModeActiveChoice=Continuous  F=60  K=1  Ts=0
  Sqrt : Sqrt  SaturateOnIntegerOverflow=on
  Sqrt1 : Sqrt  SaturateOnIntegerOverflow=on
  Sqrt2 : Sqrt  SaturateOnIntegerOverflow=on
  Total_Active_Power : Gain
  Total_Apparent_Power : Gain
  Total_RMS_Current : Gain
  Total_Reactive_Power : Gain
  measurements : Outport
  wires:
  [Current_B] -> AC_IRMS_2/1
  [P_A] -> AC_PF_1/1
  Math Function4/1 -> Add8/1
  [Voltage_A] -> Power Measurement/1
  [Current_C] -> AC_IRMS_3/1
  [Current_A] -> Power Measurement/2
  [Voltage_C] -> AC_VRMS_3/1
  Sqrt1/1 -> AC_S_2/1  "AC_S_2"
  [Voltage_B] -> AC_VRMS_2/1
  Math Function1/1 -> Add/2
  Power Measurement/2 -> AC_Q_1/1
  Math Function5/1 -> Add8/2
  [Voltage_B] -> Power Measurement1/1
  [Current_A] -> AC_IRMS_1/1
  Power Measurement/1 -> AC_P_1/1
  [Voltage_C] -> Power Measurement2/1
  Power Measurement1/2 -> AC_Q_2/1
  Add8/1 -> Sqrt2/1
  Power Measurement2/1 -> AC_P_3/1
  [Current_B] -> Power Measurement1/2
  [Q_B] -> Math Function1/1
  [P_C] -> AC_PF_3/1
  PLL (3ph)/1 -> AC_FREQ/1
  [S_C] -> AC_PF_3/2
  [P_B] -> Math Function/1
  [P_B] -> AC_PF_2/1
  [Q_A] -> Math Function3/1
  Sqrt/1 -> AC_S_1/1  "AC_S_1"
  Sqrt2/1 -> AC_S_3/1  "AC_S_3"
  [P_A] -> Math Function2/1
  Add9/1 -> Total_RMS_Current/1
  Math Function3/1 -> Add1/2
  Add1/1 -> Sqrt/1
  Math Function/1 -> Add/1
  [S_B] -> AC_PF_2/2
  [Voltage_A] -> AC_VRMS_1/1
  Power Measurement2/2 -> AC_Q_3/1
  Math Function2/1 -> Add1/1
  [Current_C] -> Power Measurement2/2
  [P_C] -> Math Function4/1
  [Q_C] -> Math Function5/1
  Add/1 -> Sqrt1/1
  Power Measurement1/1 -> AC_P_2/1
  [S_A] -> AC_PF_1/2
  RAW_MEAS/1 -> Bus Selector/1
  Bus Selector/1 -> [Voltage_A]  "<voltage_pha>"
  Bus Selector/2 -> [Voltage_B]  "<voltage_phb>"
  Bus Selector/3 -> [Voltage_C]  "<voltage_phc>"
  AC_P_2/1 -> Add2/2, Bus Creator2/2  "AC_P_2"
  AC_P_3/1 -> Bus Creator2/3, Add2/3  "AC_P_3"
  Add2/1 -> Total_Active_Power/1
  AC_Q_1/1 -> Bus Creator3/1, Add3/1  "AC_Q_1"
  AC_Q_2/1 -> Bus Creator3/2, Add3/2  "AC_Q_2"
  AC_Q_3/1 -> Bus Creator3/3, Add3/3  "AC_Q_3"
  Add3/1 -> Total_Reactive_Power/1
  Add4/1 -> Total_Apparent_Power/1
  AC_VRMS_1/1 -> Bus Creator/1  "AC_VRMS_1"
  AC_VRMS_2/1 -> Bus Creator/2  "AC_VRMS_2"
  AC_VRMS_3/1 -> Bus Creator/3  "AC_VRMS_3"
  Bus Creator/1 -> [voltage_RMS]
  AC_IRMS_1/1 -> Bus Creator1/1, Add9/1  "AC_IRMS_1"
  AC_IRMS_2/1 -> Bus Creator1/2, Add9/2  "AC_IRMS_2"
  Bus Creator1/1 -> [current_RMS]
  AC_IRMS_3/1 -> Bus Creator1/3, Add9/3  "AC_IRMS_3"
  Total_RMS_Current/1 -> Bus Creator1/4  "Total_RMS_Current"
  Total_Active_Power/1 -> Bus Creator2/4  "Total_Active_Power"
  Bus Creator2/1 -> [active_power]
  Bus Creator3/1 -> [reactive_power]
  Total_Reactive_Power/1 -> Bus Creator3/4  "Total_Reactive_Power"
  [active_power] -> Bus Selector1/1
  Bus Selector1/1 -> [P_A]  "<AC_P_1>"
  Bus Selector1/2 -> [P_B]  "<AC_P_2>"
  Bus Selector1/3 -> [P_C]  "<AC_P_3>"
  [reactive_power] -> Bus Selector2/1
  Bus Creator5/1 -> [apparent_power]
  Total_Apparent_Power/1 -> Bus Creator5/4  "Total_Apparent_Power"
  Bus Selector2/1 -> [Q_A]  "<AC_Q_1>"
  Bus Selector2/2 -> [Q_B]  "<AC_Q_2>"
  Bus Selector2/3 -> [Q_C]  "<AC_Q_3>"
  Bus Creator6/1 -> [power_factor]
  AC_PF_3/1 -> Bus Creator6/3  "AC_PF_3"
  AC_PF_1/1 -> Bus Creator6/1  "AC_PF_1"
  AC_PF_2/1 -> Bus Creator6/2  "AC_PF_2"
  [voltage_RMS] -> Bus Creator7/1  "voltage_RMS"
  [current_RMS] -> Bus Creator7/2  "current_RMS"
  [frequency] -> Bus Creator7/3  "frequency"
  [active_power] -> Bus Creator7/4  "active_power"
  [reactive_power] -> Bus Creator7/5  "reactive_power"
  [power_factor] -> Bus Creator7/6  "power_factor"
  Bus Creator7/1 -> measurements/1
  AC_S_1/1 -> Bus Creator5/1, Add4/1
  AC_S_2/1 -> Bus Creator5/2, Add4/2
  AC_S_3/1 -> Bus Creator5/3, Add4/3
  AC_P_1/1 -> Add2/1, Bus Creator2/1  "AC_P_1"
  [Voltage_A] -> Mux/1
  [Voltage_B] -> Mux/2
  [Voltage_C] -> Mux/3
  Mux/1 -> PLL (3ph)/1
  AC_FREQ/1 -> [frequency]  "AC_FREQ"
  Bus Selector/4 -> [Current_A]  "<current_pha>"
  Bus Selector/5 -> [Current_B]  "<current_phb>"
  Bus Selector/6 -> [Current_C]  "<current_phc>"

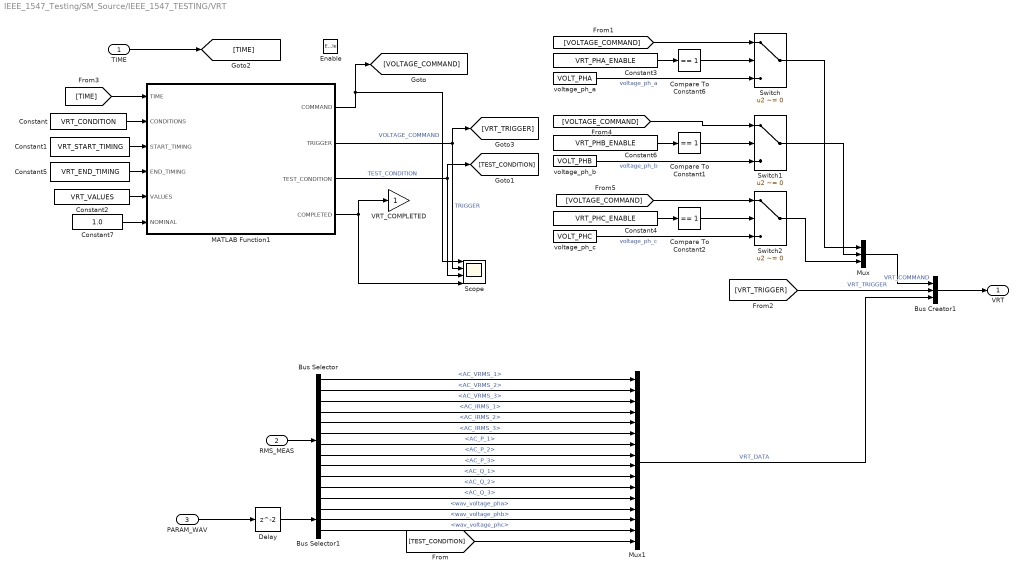
== system IEEE_1547_Testing/SM_Source/IEEE_1547_TESTING/VRT ==
  TIME : Inport
  RMS_MEAS : Inport  Port=2
  PARAM_WAV : Inport  Port=3
  Enable : EnablePort
  Bus Creator1 : BusCreator  Inputs=3
  Bus Selector : BusSelector  OutputSignals=voltage_RMS.AC_VRMS_1,voltage_RMS.AC_VRMS_2,voltage_RMS.AC_VRMS_3,current_RMS.AC_IRMS_1,current_RMS.AC_IRMS_2,current_RMS.AC_IRMS_3,active_power.AC_P_1,active_power.AC_P_2,active_power.AC_P_3,reactive_power.AC_Q_1,reactive_power.AC_Q_2,reactive_power.AC_Q_3
  Bus Selector1 : BusSelector  OutputSignals=wav_voltage_pha,wav_voltage_phb,wav_voltage_phc
  Compare To Constant1 : simulink/Logic and Bit Operations/Compare To Constant  relop===  const=1  OutDataTypeStr=boolean
  Compare To Constant2 : simulink/Logic and Bit Operations/Compare To Constant  relop===  const=1  OutDataTypeStr=boolean
  Compare To Constant6 : simulink/Logic and Bit Operations/Compare To Constant  relop===  const=1  OutDataTypeStr=boolean
  Constant : Constant  Value=VRT_CONDITION
  Constant1 : Constant  Value=VRT_START_TIMING
  Constant2 : Constant  Value=VRT_VALUES
  Constant3 : Constant  Value=VRT_PHA_ENABLE
  Constant4 : Constant  Value=VRT_PHC_ENABLE
  Constant5 : Constant  Value=VRT_END_TIMING
  Constant6 : Constant  Value=VRT_PHB_ENABLE
  Constant7 : Constant  Value=1.0
  Delay : Delay
  MATLAB Function1 : MATLAB Function  TreatAsAtomicUnit=on
  Mux : Mux  Inputs=3
  Mux1 : Mux  Inputs=16
  Scope : Scope  NumInputPorts=4
  Switch : Switch  Criteria=u2 ~= 0
  Switch1 : Switch  Criteria=u2 ~= 0
  Switch2 : Switch  Criteria=u2 ~= 0
  VRT_COMPLETED : Gain
  voltage_ph_a : Constant  Value=VOLT_PHA
  voltage_ph_b : Constant  Value=VOLT_PHB
  voltage_ph_c : Constant  Value=VOLT_PHC
  VRT : Outport  VectorParamsAs1DForOutWhenUnconnected=on
  wires:
  Bus Creator1/1 -> VRT/1
  Bus Selector/12 -> Mux1/12  "<AC_Q_3>"
  Bus Selector/9 -> Mux1/9  "<AC_P_3>"
  Bus Selector/8 -> Mux1/8  "<AC_P_2>"
  Bus Selector/7 -> Mux1/7  "<AC_P_1>"
  Bus Selector/11 -> Mux1/11  "<AC_Q_2>"
  Bus Selector/10 -> Mux1/10  "<AC_Q_1>"
  RMS_MEAS/1 -> Bus Selector/1
  PARAM_WAV/1 -> Delay/1
  Bus Selector1/1 -> Mux1/13  "<wav_voltage_pha>"
  Bus Selector1/2 -> Mux1/14  "<wav_voltage_phb>"
  Delay/1 -> Bus Selector1/1
  Mux/1 -> Bus Creator1/1  "VRT_COMMAND"
  Bus Selector/1 -> Mux1/1  "<AC_VRMS_1>"
  Bus Selector/2 -> Mux1/2  "<AC_VRMS_2>"
  Bus Selector/3 -> Mux1/3  "<AC_VRMS_3>"
  Bus Selector/4 -> Mux1/4  "<AC_IRMS_1>"
  Bus Selector/5 -> Mux1/5  "<AC_IRMS_2>"
  Bus Selector/6 -> Mux1/6  "<AC_IRMS_3>"
  MATLAB Function1/1(COMMAND) -> Scope/1, [VOLTAGE_COMMAND]  "VOLTAGE_COMMAND"
  Constant2/1 -> MATLAB Function1/5(VALUES)
  Constant1/1 -> MATLAB Function1/3(START_TIMING)
  Constant/1 -> MATLAB Function1/2(CONDITIONS)
  [TIME] -> MATLAB Function1/1(TIME)
  TIME/1 -> [TIME]
  [VRT_TRIGGER] -> Bus Creator1/2  "VRT_TRIGGER"
  Bus Selector1/3 -> Mux1/15  "<wav_voltage_phc>"
  Constant5/1 -> MATLAB Function1/4(END_TIMING)
  MATLAB Function1/2(TRIGGER) -> [VRT_TRIGGER], Scope/2  "TRIGGER"
  MATLAB Function1/3(TEST_CONDITION) -> [TEST_CONDITION], Scope/3  "TEST_CONDITION"
  MATLAB Function1/4(COMPLETED) -> VRT_COMPLETED/1, Scope/4
  [TEST_CONDITION] -> Mux1/16
  voltage_ph_a/1 -> Switch/3  "voltage_ph_a"
  [VOLTAGE_COMMAND] -> Switch/1
  Constant3/1 -> Compare To Constant6/1
  Compare To Constant6/1 -> Switch/2
  Compare To Constant1/1 -> Switch1/2
  Constant6/1 -> Compare To Constant1/1
  [VOLTAGE_COMMAND] -> Switch1/1
  voltage_ph_b/1 -> Switch1/3  "voltage_ph_b"
  voltage_ph_c/1 -> Switch2/3  "voltage_ph_c"
  [VOLTAGE_COMMAND] -> Switch2/1
  Constant4/1 -> Compare To Constant2/1
  Compare To Constant2/1 -> Switch2/2
  Switch/1 -> Mux/1
  Switch1/1 -> Mux/2
  Switch2/1 -> Mux/3
  Constant7/1 -> MATLAB Function1/6(NOMINAL)
  Mux1/1 -> Bus Creator1/3  "VRT_DATA"

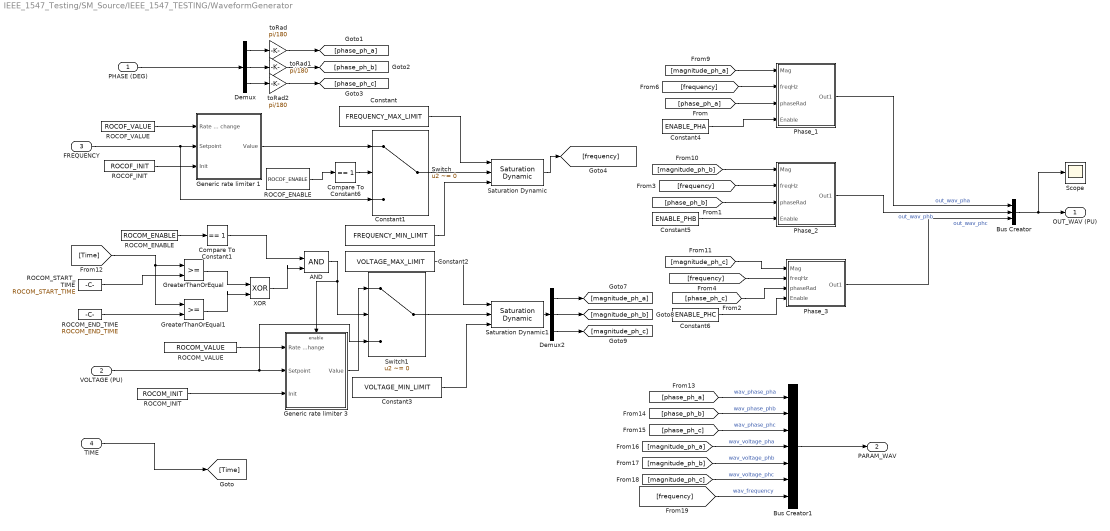
== system IEEE_1547_Testing/SM_Source/IEEE_1547_TESTING/WaveformGenerator ==
  PHASE (DEG) : Inport
  VOLTAGE (PU) : Inport  Port=2
  FREQUENCY : Inport  Port=3
  TIME : Inport  Port=4
  AND : Logic  IconShape=distinctive  AllPortsSameDT=off  OutDataTypeStr=boolean
  Bus Creator : BusCreator  Inputs=3
  Bus Creator1 : BusCreator  Inputs=7
  Compare To Constant1 : simulink/Logic and Bit Operations/Compare To Constant  relop===  const=1  OutDataTypeStr=boolean
  Compare To Constant6 : simulink/Logic and Bit Operations/Compare To Constant  relop===  const=1  OutDataTypeStr=boolean
  Constant : Constant  Value=FREQUENCY_MAX_LIMIT
  Constant1 : Constant  Value=FREQUENCY_MIN_LIMIT
  Constant2 : Constant  Value=VOLTAGE_MAX_LIMIT
  Constant3 : Constant  Value=VOLTAGE_MIN_LIMIT
  Constant4 : Constant  Value=ENABLE_PHA
  Constant5 : Constant  Value=ENABLE_PHB
  Constant6 : Constant  Value=ENABLE_PHC
  Demux : Demux  Outputs=3
  Demux2 : Demux  Outputs=3
  Generic rate limiter 1 : Subsystem
  Generic rate limiter 3 : Subsystem
  GreaterThanOrEqual : RelationalOperator  OutDataTypeStr=boolean  RndMeth=Simplest
  GreaterThanOrEqual1 : RelationalOperator  OutDataTypeStr=boolean  RndMeth=Simplest
  Phase_1 : Subsystem
  Phase_2 : Subsystem
  Phase_3 : Subsystem
  ROCOF_ENABLE : Constant  Value=ROCOF_ENABLE
  ROCOF_INIT : Constant  Value=ROCOF_INIT
  ROCOF_VALUE : Constant  Value=ROCOF_VALUE
  ROCOM_ENABLE : Constant  Value=ROCOM_ENABLE
  ROCOM_END_TIME : Constant  Value=ROCOM_END_TIME
  ROCOM_INIT : Constant  Value=ROCOM_INIT
  ROCOM_START_TIME : Constant  Value=ROCOM_START_TIME
  ROCOM_VALUE : Constant  Value=ROCOM_VALUE
  Saturation Dynamic : simulink/Discontinuities/Saturation Dynamic  OutMin=[]  OutMax=[]  OutDataTypeStr=Inherit: Same as second input  OutDataType=fixdt(1, 16)  OutScaling=2^-10  DoSatur=off
  Saturation Dynamic1 : simulink/Discontinuities/Saturation Dynamic  OutMin=[]  OutMax=[]  OutDataTypeStr=Inherit: Same as second input  OutDataType=fixdt(1, 16)  OutScaling=2^-10  DoSatur=off
  Scope : Scope
  Switch : Switch  Criteria=u2 ~= 0
  Switch1 : Switch  Criteria=u2 ~= 0
  XOR : Logic  Operator=XOR  IconShape=distinctive  AllPortsSameDT=off  OutDataTypeStr=boolean
  toRad : Gain  Gain=pi/180
  toRad1 : Gain  Gain=pi/180
  toRad2 : Gain  Gain=pi/180
  OUT_WAV (PU) : Outport  VectorParamsAs1DForOutWhenUnconnected=on
  PARAM_WAV : Outport  Port=2  VectorParamsAs1DForOutWhenUnconnected=on
  wires:
  VOLTAGE (PU)/1 -> Switch1/3, Generic rate limiter 3/2("Setpoint ")
  PHASE (DEG)/1 -> Demux/1
  Demux/1 -> toRad/1
  Demux/2 -> toRad1/1
  Demux/3 -> toRad2/1
  [phase_ph_a] -> Phase_1/3(phaseRad)
  [phase_ph_b] -> Phase_2/3(phaseRad)
  [phase_ph_c] -> Phase_3/3(phaseRad)
  Generic rate limiter 1/1(Value) -> Switch/1
  FREQUENCY/1 -> Switch/3, Generic rate limiter 1/2("Setpoint ")
  ROCOF_VALUE/1 -> Generic rate limiter 1/1(Rate of change)
  ROCOF_INIT/1 -> Generic rate limiter 1/3(Init)
  ROCOF_ENABLE/1 -> Compare To Constant6/1
  Compare To Constant6/1 -> Switch/2
  ROCOM_VALUE/1 -> Generic rate limiter 3/1(Rate of change)
  ROCOM_INIT/1 -> Generic rate limiter 3/3(Init)
  [frequency] -> Phase_1/2(freqHz)
  [frequency] -> Phase_2/2(freqHz)
  Demux2/1 -> [magnitude_ph_a]
  Demux2/2 -> [magnitude_ph_b]
  Demux2/3 -> [magnitude_ph_c]
  [magnitude_ph_a] -> Phase_1/1(Mag)
  [magnitude_ph_b] -> Phase_2/1(Mag)
  [magnitude_ph_c] -> Phase_3/1(Mag)
  [Time] -> GreaterThanOrEqual1/1, GreaterThanOrEqual/1
  ROCOM_START_TIME/1 -> GreaterThanOrEqual/2
  ROCOM_END_TIME/1 -> GreaterThanOrEqual1/2
  GreaterThanOrEqual/1 -> XOR/1
  GreaterThanOrEqual1/1 -> XOR/2
  Switch1/1 -> Saturation Dynamic1/2
  Generic rate limiter 3/1(Value) -> Switch1/1
  AND/1 -> Switch1/2, Generic rate limiter 3/Enable
  XOR/1 -> AND/2
  Compare To Constant1/1 -> AND/1
  ROCOM_ENABLE/1 -> Compare To Constant1/1
  Switch/1 -> Saturation Dynamic/2
  TIME/1 -> [Time]
  Phase_1/1(Out1) -> Bus Creator/1  "out_wav_pha"
  Phase_2/1(Out1) -> Bus Creator/2  "out_wav_phb"
  Phase_3/1(Out1) -> Bus Creator/3  "out_wav_phc"
  Bus Creator/1 -> Scope/1, OUT_WAV (PU)/1
  [phase_ph_a] -> Bus Creator1/1  "wav_phase_pha"
  [phase_ph_b] -> Bus Creator1/2  "wav_phase_phb"
  [phase_ph_c] -> Bus Creator1/3  "wav_phase_phc"
  [magnitude_ph_a] -> Bus Creator1/4  "wav_voltage_pha"
  [magnitude_ph_b] -> Bus Creator1/5  "wav_voltage_phb"
  [magnitude_ph_c] -> Bus Creator1/6  "wav_voltage_phc"
  [frequency] -> Bus Creator1/7  "wav_frequency"
  Bus Creator1/1 -> PARAM_WAV/1
  Saturation Dynamic/1 -> [frequency]
  Saturation Dynamic1/1 -> Demux2/1
  Constant/1 -> Saturation Dynamic/1
  Constant1/1 -> Saturation Dynamic/3
  Constant2/1 -> Saturation Dynamic1/1
  Constant3/1 -> Saturation Dynamic1/3
  toRad/1 -> [phase_ph_a]
  toRad1/1 -> [phase_ph_b]
  toRad2/1 -> [phase_ph_c]
  Constant4/1 -> Phase_1/4(Enable)
  Constant5/1 -> Phase_2/4(Enable)
  [frequency] -> Phase_3/2(freqHz)
  Constant6/1 -> Phase_3/4(Enable)

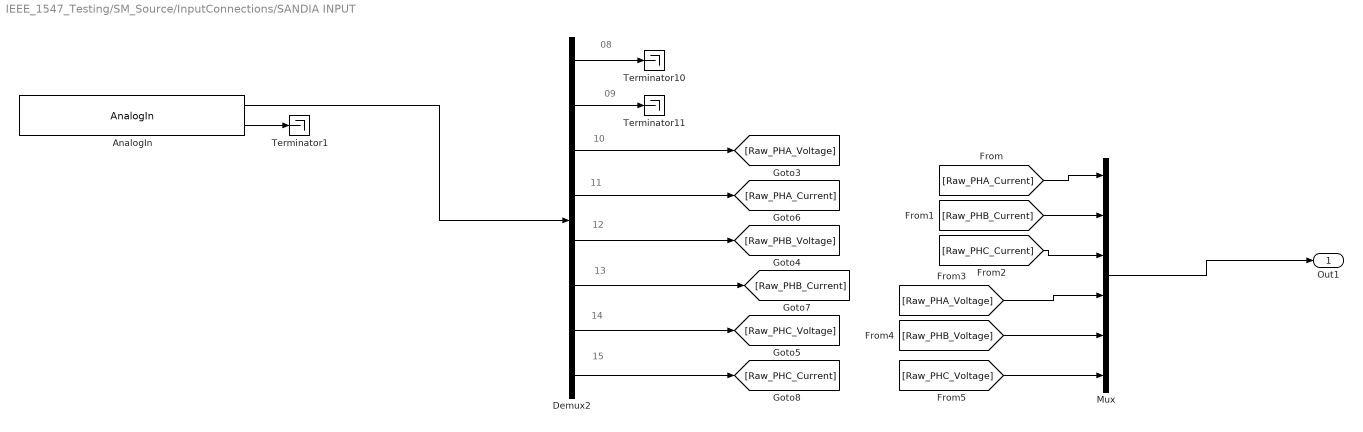
== system IEEE_1547_Testing/SM_Source/InputConnections/SANDIA INPUT ==
  note: 11
  note: 14
  note: 09
  note: 12
  note: 13
  note: 15
  note: 08
  note: 10
  AnalogIn : rtio_opalrt_common/AnalogIn  CtrlName='OpCtrl'  portNb=2  FcnNos=Slot 1 Module B Subsection 2  size=16  maxcount=8  count=8  numchan=8  sampleTime=0
      settings: AttributesFormatString=%<CtrlName>
  Demux2 : Demux  Outputs=8
  Mux : Mux  Inputs=6
  Terminator1 : Terminator
  Terminator10 : Terminator
  Terminator11 : Terminator
  Out1 : Outport
  wires:
  Demux2/2 -> Terminator11/1
  Demux2/1 -> Terminator10/1
  Demux2/6 -> [Raw_PHB_Current]
  Demux2/7 -> [Raw_PHC_Voltage]
  Demux2/8 -> [Raw_PHC_Current]
  Demux2/3 -> [Raw_PHA_Voltage]
  Demux2/5 -> [Raw_PHB_Voltage]
  Demux2/4 -> [Raw_PHA_Current]
  Mux/1 -> Out1/1
  [Raw_PHC_Current] -> Mux/3
  [Raw_PHA_Voltage] -> Mux/4
  [Raw_PHC_Voltage] -> Mux/6
  [Raw_PHA_Current] -> Mux/1
  [Raw_PHB_Voltage] -> Mux/5
  [Raw_PHB_Current] -> Mux/2
  AnalogIn/1 -> Demux2/1
  AnalogIn/2 -> Terminator1/1

== system IEEE_1547_Testing/SM_Source/IEEE_1547_TESTING/DataAcquisitionSystem/Subsystem ==
  In1 : Inport
  Enable : EnablePort
  FILE_LIMIT : Gain
  FILE_STATUS : Gain
  OpWriteFile : rtlab/DataLogging/OpWriteFile  Static_File=on  varname=Data  Filename=Data.mat  rtpath='./'  nrtpath='.\'  Acq_Group=28  file_size=1e+8  write_offline=off  Sim_Mode=off  Nb_Samples=500  Buffer_size=200000
      settings: SourceProductName=RT-LAB  Decimation=25
  Terminator : Terminator
  Terminator1 : Terminator
  wires:
  OpWriteFile/1 -> FILE_LIMIT/1
  FILE_LIMIT/1 -> Terminator/1
  OpWriteFile/2 -> FILE_STATUS/1
  FILE_STATUS/1 -> Terminator1/1
  In1/1 -> OpWriteFile/1

== system IEEE_1547_Testing/SM_Source/IEEE_1547_TESTING/DataAcquisitionSystem/Subsystem1 ==
  In1 : Inport
  Enable : EnablePort
  FILE_LIMIT : Gain
  FILE_STATUS : Gain
  OpWriteFile : rtlab/DataLogging/OpWriteFile  Static_File=on  varname=Data  Filename=WAV.mat  rtpath='./'  nrtpath='.\'  Acq_Group=27  file_size=3e+8  write_offline=off  Sim_Mode=off  Nb_Samples=1000  Buffer_size=200000
      settings: SourceProductName=RT-LAB  Decimation=4
  Terminator : Terminator
  Terminator1 : Terminator
  wires:
  In1/1 -> OpWriteFile/1
  FILE_STATUS/1 -> Terminator1/1
  OpWriteFile/2 -> FILE_STATUS/1
  FILE_LIMIT/1 -> Terminator/1
  OpWriteFile/1 -> FILE_LIMIT/1
